simulink model "MasseMitFeder"  (R2023b)
settings: Solver=ode1  StartTime=0.0  StopTime=10.0  FixedStep=0.00001  RelTol=1e-3
settings Model: Creator=PM  LastModifiedBy=PM

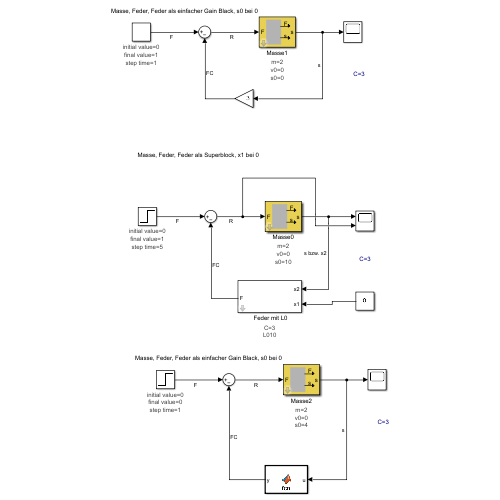
[thumbnail: Simulink's stored preview of the top-level diagram]
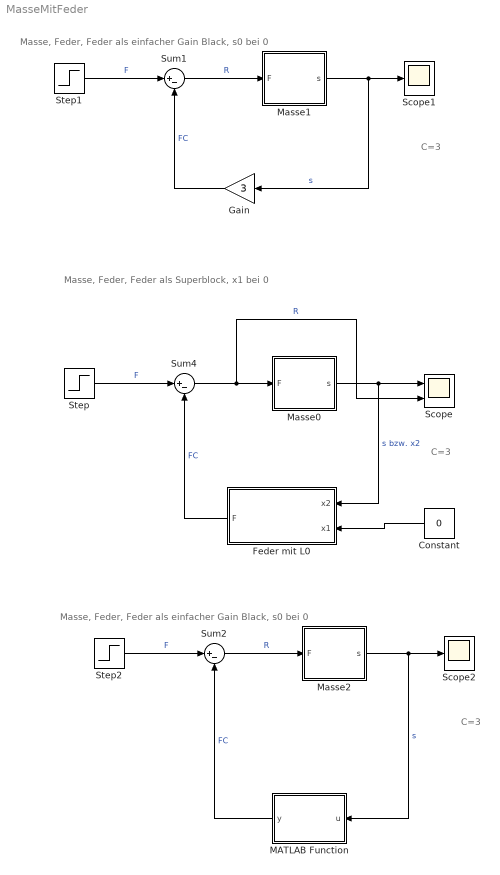
== system MasseMitFeder ==
  note: Masse, Feder, Feder als einfacher Gain Black, s0 bei 0
  note: C=3
  note: C=3
  note: Masse, Feder, Feder als Superblock, x1 bei 0
  note: C=3
  note: Masse, Feder, Feder als einfacher Gain Black, s0 bei 0
  " Feder mit L0" : Subsystem  mask{C=3, L0=10}
      mask prompts: C "Spring Constant C [N/m]"; L0 "Length of Spring if no force is applied L0 [m]"
      mask help:
      | If no force F is applied, the spring has the length L0.
      |
      | F=C*sign(x2-x1-L0)*((x2-x1-L0)
      settings: AttributesFormatString=|
      | C=%<C>
      | L0%<L0>
  Constant : Constant  Value=0
  Gain : Gain  Gain=3
  MATLAB Function : MATLAB Function  TreatAsAtomicUnit=on
  Masse0 : Subsystem  mask(Starrer Körper){m=2, v0=0, s0=10}
      mask prompts: m "Masse m"; v0 "Anfangsgeschwindigkeit v0"; s0 "Anfangsposition s0"
      mask help: Berechnet die Position eines Körpers als Funktion der auf ihn wirkenden Kraft F, seiner Masse m, der Anfangsgeschwindigkeit v0 und der Anfangsposition s0.
      settings: AttributesFormatString=m=%<m>\nv0=%<v0>\ns0=%<s0>
      mask Help:
      | Die Position x eines starren Körpers der Masse m berechnet sich aus:
      | F=m*X''
      | 
      | Erstellt von Patrick Metzler für Hochschule RheinMain.
      mask Display:
      | plot(0,0)
      | plot(100,100)
      | patch([20 20 60 60],[10 90 90 10],[0.7,0.7,0.7])
      | plot([60 80],[70 70])
      | patch([80 80 85],[65 75 70],[0 0 0])
      | text(70,80,'F')
      | plot([60 80],[30 30])
      | patch([80 80 85],[25 35 30],[0 0 0])
      | text(70,40,'s')
      | port_label ('output',1,'s')
      | port_label ('input',1,'F')
  Masse1 : Subsystem  mask(Starrer Körper){m=2, v0=0, s0=0}
      mask prompts: m "Masse m"; v0 "Anfangsgeschwindigkeit v0"; s0 "Anfangsposition s0"
      mask help: Berechnet die Position eines Körpers als Funktion der auf ihn wirkenden Kraft F, seiner Masse m, der Anfangsgeschwindigkeit v0 und der Anfangsposition s0.
      settings: AttributesFormatString=m=%<m>\nv0=%<v0>\ns0=%<s0>
      mask Help:
      | Die Position x eines starren Körpers der Masse m berechnet sich aus:
      | F=m*X''
      | 
      | Erstellt von Patrick Metzler für Hochschule RheinMain.
      mask Display:
      | plot(0,0)
      | plot(100,100)
      | patch([20 20 60 60],[10 90 90 10],[0.7,0.7,0.7])
      | plot([60 80],[70 70])
      | patch([80 80 85],[65 75 70],[0 0 0])
      | text(70,80,'F')
      | plot([60 80],[30 30])
      | patch([80 80 85],[25 35 30],[0 0 0])
      | text(70,40,'s')
      | port_label ('output',1,'s')
      | port_label ('input',1,'F')
  Masse2 : Subsystem  mask(Starrer Körper){m=2, v0=0, s0=4}
      mask prompts: m "Masse m"; v0 "Anfangsgeschwindigkeit v0"; s0 "Anfangsposition s0"
      mask help: Berechnet die Position eines Körpers als Funktion der auf ihn wirkenden Kraft F, seiner Masse m, der Anfangsgeschwindigkeit v0 und der Anfangsposition s0.
      settings: AttributesFormatString=m=%<m>\nv0=%<v0>\ns0=%<s0>
      mask Help:
      | Die Position x eines starren Körpers der Masse m berechnet sich aus:
      | F=m*X''
      | 
      | Erstellt von Patrick Metzler für Hochschule RheinMain.
      mask Display:
      | plot(0,0)
      | plot(100,100)
      | patch([20 20 60 60],[10 90 90 10],[0.7,0.7,0.7])
      | plot([60 80],[70 70])
      | patch([80 80 85],[65 75 70],[0 0 0])
      | text(70,80,'F')
      | plot([60 80],[30 30])
      | patch([80 80 85],[25 35 30],[0 0 0])
      | text(70,40,'s')
      | port_label ('output',1,'s')
      | port_label ('input',1,'F')
  Scope : Scope  NumInputPorts=2
  Scope1 : Scope
  Scope2 : Scope
  Step : Step  Time=5  SampleTime=0
      settings: AttributesFormatString=initial value=%<Before>\nfinal value=%<After>\nstep time=%<Time>
  Step1 : Step  SampleTime=0
      settings: AttributesFormatString=initial value=%<Before>\nfinal value=%<After>\nstep time=%<Time>
  Step2 : Step  After=0  SampleTime=0
      settings: AttributesFormatString=initial value=%<Before>\nfinal value=%<After>\nstep time=%<Time>
  Sum1 : Sum  Inputs=|+-
  Sum2 : Sum  Inputs=|+-
  Sum4 : Sum  Inputs=|+-
  wires:
  Step/1 -> Sum4/1  "F"
  Sum4/1 -> Scope/2, Masse0/1(F)  "R"
  Masse0/1(s) -> Scope/1, " Feder mit L0"/1(x2)  "s bzw. x2"
  " Feder mit L0"/1(F) -> Sum4/2  "FC"
  Constant/1 -> " Feder mit L0"/2(x1)
  Gain/1 -> Sum1/2  "FC"
  Sum1/1 -> Masse1/1(F)  "R"
  Step1/1 -> Sum1/1  "F"
  Masse1/1(s) -> Scope1/1, Gain/1  "s"
  MATLAB Function/1(y) -> Sum2/2  "FC"
  Sum2/1 -> Masse2/1(F)  "R"
  Step2/1 -> Sum2/1  "F"
  Masse2/1(s) -> MATLAB Function/1(u), Scope2/1  "s"

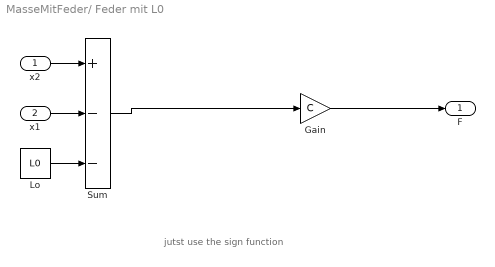
== system MasseMitFeder/ Feder mit L0 ==
  note: jutst use the sign function
  x2 : Inport
  x1 : Inport  Port=2
  Gain : Gain  Gain=C
  Lo : Constant  Value=L0
  Sum : Sum  Inputs=+--
  F : Outport  VectorParamsAs1DForOutWhenUnconnected=off
  wires:
  x2/1 -> Sum/1
  x1/1 -> Sum/2
  Lo/1 -> Sum/3
  Sum/1 -> Gain/1
  Gain/1 -> F/1

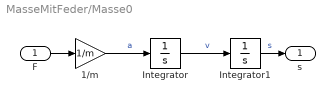
== system MasseMitFeder/Masse0 ==
  F : Inport
  1/m : Gain  Gain=1/m
  Integrator : Integrator  InitialCondition=v0
  Integrator1 : Integrator  InitialCondition=s0
  s : Outport  VectorParamsAs1DForOutWhenUnconnected=off
  wires:
  Integrator1/1 -> s/1  "s"
  F/1 -> 1/m/1
  Integrator/1 -> Integrator1/1  "v"
  1/m/1 -> Integrator/1  "a"

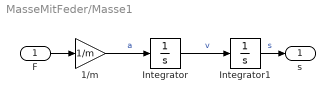
== system MasseMitFeder/Masse1 ==
  F : Inport
  1/m : Gain  Gain=1/m
  Integrator : Integrator  InitialCondition=v0
  Integrator1 : Integrator  InitialCondition=s0
  s : Outport  VectorParamsAs1DForOutWhenUnconnected=off
  wires:
  Integrator1/1 -> s/1  "s"
  F/1 -> 1/m/1
  Integrator/1 -> Integrator1/1  "v"
  1/m/1 -> Integrator/1  "a"

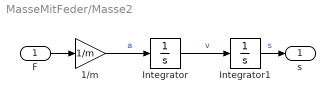
== system MasseMitFeder/Masse2 ==
  F : Inport
  1/m : Gain  Gain=1/m
  Integrator : Integrator  InitialCondition=v0
  Integrator1 : Integrator  InitialCondition=s0
  s : Outport  VectorParamsAs1DForOutWhenUnconnected=off
  wires:
  Integrator1/1 -> s/1  "s"
  F/1 -> 1/m/1
  Integrator/1 -> Integrator1/1  "v"
  1/m/1 -> Integrator/1  "a"

== matlab function MasseMitFeder/MATLAB Function ==
  data: u input; y output
function y = fcn(u)
if u>0
y = 3*u;
else
y=-1000;
%y = 3*u;
end
